simulink model "rtwdemo_whilesl"  (Simulink 7.1)
settings: Solver=FixedStepDiscrete  StartTime=0.0  StopTime=10.0  FixedStep=.01  RelTol=1e-3
settings Model: Creator=ajayaram  LastModifiedBy=ajayaram
settings OptimizationCC: InlineParams=on  InlineInvariantSignals=on  OptimizeModelRefInitCode=on  LifeSpan=1
settings DebuggingCC: SaveWithParameterizedLinksMsg=none  StrictBusMsg=ErrorLevel1
settings RTWCC: SystemTargetFile=ert.tlc  GenCodeOnly=on  GenerateMakefile=off  TemplateMakefile=ert_default_tmf  Description=Real-Time Workshop Embedded Coder (no auto configuration)  GenerateReport=on  ProcessScript=ert_make_rtw_hook  IncludeHyperlinkInReport=on  LaunchReport=on
settings CodeAppCC: GenerateComments=off  IgnoreCustomStorageClasses=off  SimulinkBlockComments=off
settings ERTTargetCC: TargetFcnLib=ansi_tfl_tmw.mat  GenerateSampleERTMain=on  InlinedParameterPlacement=NonHierarchical  ERTCustomFileTemplate=example_file_process.tlc

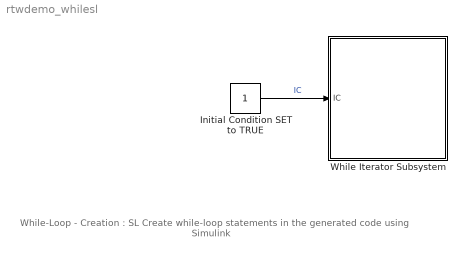
== system rtwdemo_whilesl ==
  note: While-Loop - Creation : SL
      | Create while-loop statements in the
      | generated code using Simulink
  Initial Condition SET to TRUE : Constant  OutDataTypeMode=boolean  OutDataType=sfix(16)  OutScaling=2^0  OutDataTypeStr=boolean
  While Iterator Subsystem : Subsystem  TreatAsAtomicUnit=on
  wires:
  Initial Condition SET to TRUE/1 -> While Iterator Subsystem/1(IC)  "IC"

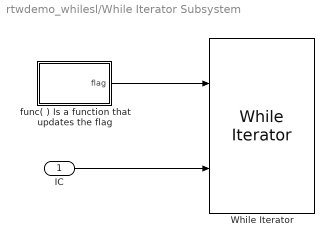
== system rtwdemo_whilesl/While Iterator Subsystem ==
  IC : Inport  OutDataType=sfix(16)  OutScaling=2^0
  While Iterator : WhileIterator  MaxIters=100  ResetStates=reset
  func( ) Is a function that updates the flag : Subsystem  TreatAsAtomicUnit=on  RTWFcnName=func  RTWFileName=whilesl
      settings: RTWSystemCode=Function  RTWFcnNameOpts=User specified
  wires:
  IC/1 -> While Iterator/2
  func( ) Is a function that updates the flag/1(flag) -> While Iterator/1

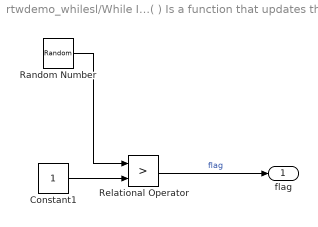
== system rtwdemo_whilesl/While Iterator Subsystem/func( ) Is a function that updates the flag ==
  Constant1 : Constant  OutDataTypeMode=boolean  OutDataType=sfix(16)  OutScaling=2^0  OutDataTypeStr=boolean
  Random Number : RandomNumber  Variance=3
  Relational Operator : RelationalOperator  Operator=>  LogicOutDataTypeMode=boolean  OutDataTypeStr=boolean
  flag : Outport  OutDataType=sfix(16)  OutScaling=2^0
  wires:
  Constant1/1 -> Relational Operator/2
  Relational Operator/1 -> flag/1  "flag"
  Random Number/1 -> Relational Operator/1
